simulink model "rle_simu"  (R2023b)
settings: Solver=VariableStepAuto  StartTime=0.0  StopTime=10.0  RelTol=1e-3
settings SFSimCC: SimTargetLang=C++

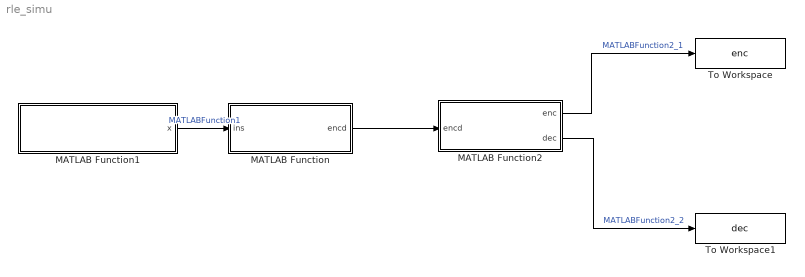
== system rle_simu ==
  MATLAB Function : MATLAB Function  TreatAsAtomicUnit=on
  MATLAB Function1 : MATLAB Function  TreatAsAtomicUnit=on
  MATLAB Function2 : MATLAB Function  TreatAsAtomicUnit=on
  To Workspace : ToWorkspace  VariableName=enc  SaveFormat=Timeseries  SampleTime=-1
      settings: Save2DSignal=2-D array (concatenate along first dimension)
  To Workspace1 : ToWorkspace  VariableName=dec  SaveFormat=Structure  SampleTime=-1
      settings: Save2DSignal=2-D array (concatenate along first dimension)
  wires:
  MATLAB Function1/1(x) -> MATLAB Function/1(ins)  "MATLABFunction1"
  MATLAB Function/1(encd) -> MATLAB Function2/1(encd)
  MATLAB Function2/2(dec) -> To Workspace1/1  "MATLABFunction2_2"
  MATLAB Function2/1(enc) -> To Workspace/1  "MATLABFunction2_1"

== matlab function rle_simu/MATLAB Function ==
  data: ins input; encd output
function encd = rleenc(ins)


indx = find(ins);
len = length(indx);

ocnt = 1;
zcnt = 0;

enc = [];
strt = 0;


for i=1:len-1
    if(indx(1)>1 && strt==0)
        zcnt = indx(1)-1;
        enc = [enc; 0, zcnt];
        zcnt = 0;
        strt = 1;
    end

    if(indx(i+1)-indx(i)==1)
        ocnt = ocnt+1;
        up=0;
    else
        zcnt = indx(i+1) - indx(i) - 1;
        enc = [enc; 1, ocnt; 0, zcnt];
        ocnt = 1;
        zcnt = 0;
        up = 1;
    end

    if(up==0 && i == len-1)
        enc = [enc; 1, ocnt ];
    end
end
encd = enc;
end

== matlab function rle_simu/MATLAB Function2 ==
  data: enc output double; encd input double; dec output double
function [enc,dec] = rledec(encd)
enc = encd;
encd = encd';
encd = encd(:);
len = length(encd);

dec = [];

for i=1:2:len
    dec  = [dec, (ones(1,encd(i+1)))*encd(i)];
end
fprintf('RLE output:');
enc
fprintf('DEC output:');
dec
end

== matlab function rle_simu/MATLAB Function1 ==
  data: x output
function x = binary_sequence()
    x = [0 0 1 1 1 0 1 0 0 0 1 1];
    disp(['Binary Input Sequence: ',num2str(x)]);
end
